simulink model "mcb_pmsm_foc_qep_dyno_f28069m_RAMP_ON_TARGET_R2021b"  (R2021b)
settings: Solver=FixedStepDiscrete  StartTime=0.0  StopTime=4  RelTol=1e-3  EnableMultiTasking=on
InitFcn:
  | mcb_pmsm_foc_qep_dyno_f28069m_data;
undefined symbols (not defined in the file): BaseRPM, DiscIntNeverNeededParam, Down, GPTRIP1SEL, GPTRIP2SEL, inverter_motor1, inverter_motor2, PI_params_motor1, PI_params_motor2, pmsm_motor1, pmsm_motor2, PU_System_motor2, target, Ts, Ts_motor, Ts_speed, TZ1, TZ2, Up
libraries: c2802xlib x10, simulink x10, mcbcontrolslib x8, c280xlib x8, mcbpositiondecoderlib x6, c2806xlib x5, svdschedulerlib x3, autolibpmsmexterior x2, mcbplantlib x2, demo_controls x1, hdlsllib x1, slpidlib x1
(part 2 of 3)

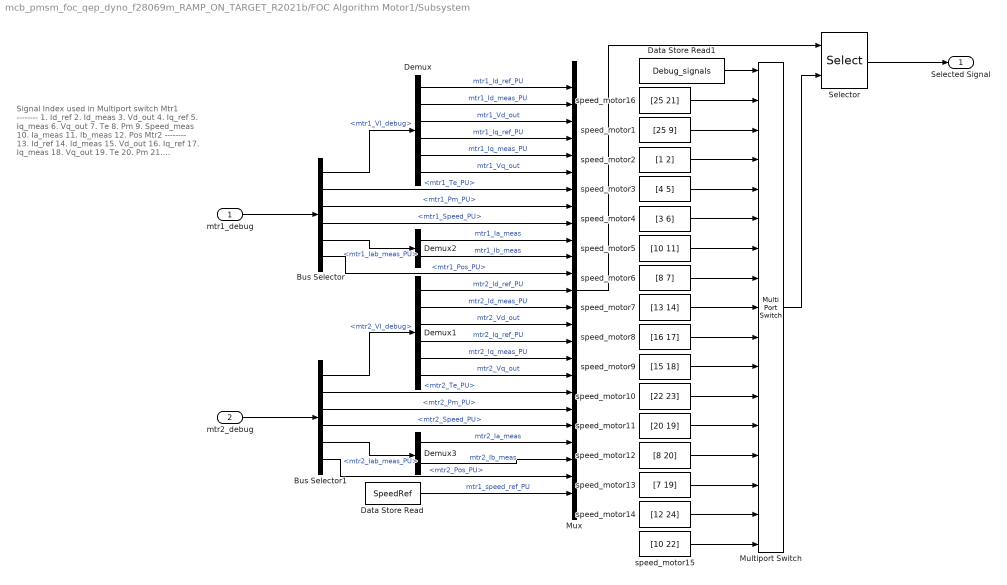
== system mcb_pmsm_foc_qep_dyno_f28069m_RAMP_ON_TARGET_R2021b/FOC Algorithm Motor1/Subsystem ==
  note: Signal Index used in Multiport switch
      | Mtr1
      | --------
      | 1. Id_ref
      | 2. Id_meas
      | 3. Vd_out
      | 4. Iq_ref
      | 5. Iq_meas
      | 6. Vq_out
      | 7. Te
      | 8. Pm
      | 9. Speed_meas
      | 10. Ia_meas
      | 11. Ib_meas
      | 12. Pos
      |
      | Mtr2
      | --------
      | 13. Id_ref
      | 14. Id_meas
      | 15. Vd_out
      | 16. Iq_ref
      | 17. Iq_meas
      | 18. Vq_out
      | 19. Te
      | 20. Pm
      | 21. Speed_meas
      | 22. Ia_meas
      | 23. Ib_meas
      | 24. Pos
      |
      | 25.Speed ref
  mtr1_debug : Inport
  mtr2_debug : Inport  Port=2
  Bus Selector : BusSelector  OutputSignals=mtr1_VI_debug,mtr1_Te_PU,mtr1_Pm_PU,mtr1_Speed_PU,mtr1_Iab_meas_PU,mtr1_Pos_PU
  Bus Selector1 : BusSelector  OutputSignals=mtr2_VI_debug,mtr2_Te_PU,mtr2_Pm_PU,mtr2_Speed_PU,mtr2_Iab_meas_PU,mtr2_Pos_PU
  Data Store Read : DataStoreRead  DataStoreName=SpeedRef  IndexOptions=Index vector (dialog)  Indices=1  OutputSizes=1
  Data Store Read1 : DataStoreRead  DataStoreName=Debug_signals  IndexOptions=Index vector (dialog)  Indices=1  OutputSizes=1
  Demux : Demux  Outputs=6
  Demux1 : Demux  Outputs=6
  Demux2 : Demux  Outputs=2
  Demux3 : Demux  Outputs=2
  Multiport Switch : MultiPortSwitch  DataPortOrder=Zero-based contiguous  Inputs=16  DiagnosticForDefault=Warning  zeroidx=on  OutDataTypeStr=uint16  RndMeth=Simplest
  Mux : Mux  Inputs=25
  Selector : Selector  InputPortWidth=25  IndexOptions=Index vector (port)  Indices=[1 3]  OutputSizes=1
  speed_motor1 : Constant  Value=[25 9]  OutDataTypeStr=uint16  SampleTime=-1
  speed_motor10 : Constant  Value=[22 23]  OutDataTypeStr=uint16  SampleTime=-1
  speed_motor11 : Constant  Value=[20 19]  OutDataTypeStr=uint16  SampleTime=-1
  speed_motor12 : Constant  Value=[8 20]  OutDataTypeStr=uint16  SampleTime=-1
  speed_motor13 : Constant  Value=[7 19]  OutDataTypeStr=uint16  SampleTime=-1
  speed_motor14 : Constant  Value=[12 24]  OutDataTypeStr=uint16  SampleTime=-1
  speed_motor15 : Constant  Value=[10 22]  OutDataTypeStr=uint16  SampleTime=-1
  speed_motor16 : Constant  Value=[25 21]  OutDataTypeStr=uint16  SampleTime=-1
  speed_motor2 : Constant  Value=[1 2]  OutDataTypeStr=uint16  SampleTime=-1
  speed_motor3 : Constant  Value=[4 5]  OutDataTypeStr=uint16  SampleTime=-1
  speed_motor4 : Constant  Value=[3 6]  OutDataTypeStr=uint16  SampleTime=-1
  speed_motor5 : Constant  Value=[10 11]  OutDataTypeStr=uint16  SampleTime=-1
  speed_motor6 : Constant  Value=[8 7]  OutDataTypeStr=uint16  SampleTime=-1
  speed_motor7 : Constant  Value=[13 14]  OutDataTypeStr=uint16  SampleTime=-1
  speed_motor8 : Constant  Value=[16 17]  OutDataTypeStr=uint16  SampleTime=-1
  speed_motor9 : Constant  Value=[15 18]  OutDataTypeStr=uint16  SampleTime=-1
  Selected Signal : Outport
  wires:
  mtr1_debug/1 -> Bus Selector/1
  mtr2_debug/1 -> Bus Selector1/1
  Bus Selector/1 -> Demux/1  "<mtr1_VI_debug>"
  Bus Selector1/1 -> Demux1/1  "<mtr2_VI_debug>"
  Demux/1 -> Mux/1  "mtr1_Id_ref_PU"
  Demux/2 -> Mux/2  "mtr1_Id_meas_PU"
  Demux/3 -> Mux/3  "mtr1_Vd_out"
  Demux/4 -> Mux/4  "mtr1_Iq_ref_PU"
  Demux/5 -> Mux/5  "mtr1_Iq_meas_PU"
  Demux/6 -> Mux/6  "mtr1_Vq_out"
  Bus Selector/2 -> Mux/7  "<mtr1_Te_PU>"
  Bus Selector/3 -> Mux/8  "<mtr1_Pm_PU>"
  Bus Selector/4 -> Mux/9  "<mtr1_Speed_PU>"
  Bus Selector/5 -> Demux2/1  "<mtr1_Iab_meas_PU>"
  Bus Selector/6 -> Mux/12  "<mtr1_Pos_PU>"
  Demux1/1 -> Mux/13  "mtr2_Id_ref_PU"
  Demux1/2 -> Mux/14  "mtr2_Id_meas_PU"
  Demux1/3 -> Mux/15  "mtr2_Vd_out"
  Demux1/4 -> Mux/16  "mtr2_Iq_ref_PU"
  Demux1/5 -> Mux/17  "mtr2_Iq_meas_PU"
  Demux1/6 -> Mux/18  "mtr2_Vq_out"
  Bus Selector1/2 -> Mux/19  "<mtr2_Te_PU>"
  Bus Selector1/3 -> Mux/20  "<mtr2_Pm_PU>"
  Bus Selector1/4 -> Mux/21  "<mtr2_Speed_PU>"
  Bus Selector1/5 -> Demux3/1  "<mtr2_Iab_meas_PU>"
  Bus Selector1/6 -> Mux/24  "<mtr2_Pos_PU>"
  Data Store Read/1 -> Mux/25  "mtr1_speed_ref_PU"
  Mux/1 -> Selector/1
  Data Store Read1/1 -> Multiport Switch/1
  Multiport Switch/1 -> Selector/2
  Selector/1 -> Selected Signal/1
  Demux2/1 -> Mux/10  "mtr1_Ia_meas"
  Demux2/2 -> Mux/11  "mtr1_Ib_meas"
  Demux3/1 -> Mux/22  "mtr2_Ia_meas"
  Demux3/2 -> Mux/23  "mtr2_Ib_meas"
  speed_motor1/1 -> Multiport Switch/3
  speed_motor2/1 -> Multiport Switch/4
  speed_motor3/1 -> Multiport Switch/5
  speed_motor4/1 -> Multiport Switch/6
  speed_motor5/1 -> Multiport Switch/7
  speed_motor6/1 -> Multiport Switch/8
  speed_motor7/1 -> Multiport Switch/9
  speed_motor8/1 -> Multiport Switch/10
  speed_motor9/1 -> Multiport Switch/11
  speed_motor10/1 -> Multiport Switch/12
  speed_motor11/1 -> Multiport Switch/13
  speed_motor12/1 -> Multiport Switch/14
  speed_motor13/1 -> Multiport Switch/15
  speed_motor14/1 -> Multiport Switch/16
  speed_motor15/1 -> Multiport Switch/17
  speed_motor16/1 -> Multiport Switch/2

== system mcb_pmsm_foc_qep_dyno_f28069m_RAMP_ON_TARGET_R2021b/FOC Algorithm Motor2/Control_System ==
  Iab_meas_PU : Inport
  Pos_PU : Inport  Port=2
  EnClosedLoop : Inport  Port=3
  Idq_ref_PU : Inport  Port=4
  Closed loop : Subsystem
  Constant : Constant  Value=0  OutDataTypeStr=dataType
  Mux1 : Mux  Inputs=3
  Switch : Switch  Criteria=u2 > Threshold  Threshold=0.5
  Duty_Cycles : Outport  VectorParamsAs1DForOutWhenUnconnected=off
  Out2 : Outport  Port=2
  wires:
  EnClosedLoop/1 -> Closed loop/4(EnablePWM), Closed loop/Enable, Switch/2
  Switch/1 -> Duty_Cycles/1
  Idq_ref_PU/1 -> Closed loop/3(Idq_ref_PU)
  Pos_PU/1 -> Closed loop/2(Pos_PU)
  Iab_meas_PU/1 -> Closed loop/1(Iab_meas_PU)
  Mux1/1 -> Switch/3
  Constant/1 -> Mux1/3, Mux1/2, Mux1/1
  Closed loop/1(Vabc in PU) -> Switch/1
  Closed loop/2(Idq_debug) -> Out2/1

== system mcb_pmsm_foc_qep_dyno_f28069m_RAMP_ON_TARGET_R2021b/FOC Algorithm Motor2/Enable Motor2 after a delay ==
  Delay to start motor1 (codegen) : Subsystem  TreatAsAtomicUnit=on  VariantControl=(codegen)
  Delay to start motor2 (sim) : Subsystem  VariantControl=(sim)

== system mcb_pmsm_foc_qep_dyno_f28069m_RAMP_ON_TARGET_R2021b/FOC Algorithm Motor2/HW_Inputs1 ==
  Sim : Inport
  Sensor Driver Blocks (codegen) : Subsystem  VariantControl=(codegen)
  Sensor Driver Blocks (sim) : Subsystem  VariantControl=(sim)
  out : Outport

== system mcb_pmsm_foc_qep_dyno_f28069m_RAMP_ON_TARGET_R2021b/FOC Algorithm Motor2/Input Scaling ==
  note: Current Measurements
  Ia_ADC : Inport
  Ib_ADC : Inport  Port=2
  QEP_Position_Count : Inport  Port=3
  QEP_Index_Latch : Inport  Port=4
  " Calculate Speed" : Subsystem
  Calculate Phase Currents : Subsystem
  Constant : Constant  Value=pmsm_motor2.PositionOffset  OutDataTypeStr=dataType  SampleTime=-1
  speed_PU : Outport
  Iab_meas_PU : Outport  Port=2
  Pos_PU : Outport  Port=3
  EnClosedLoop : Outport  Port=4
  wires:
  " Calculate Speed"/2(speed) -> speed_PU/1
  Calculate Phase Currents/1(Iab_meas_PU) -> Iab_meas_PU/1  "Iab_fb_PU"
  QEP_Position_Count/1 -> " Calculate Speed"/1(QEP_Position_Count)
  " Calculate Speed"/1(Theta_e) -> Pos_PU/1
  Ia_ADC/1 -> Calculate Phase Currents/1(Ia_ADC)
  Ib_ADC/1 -> Calculate Phase Currents/2(Ib_ADC)
  Constant/1 -> " Calculate Speed"/3(Offset)
  QEP_Index_Latch/1 -> " Calculate Speed"/2(QEP_Index_Latch)
  " Calculate Speed"/3(IndexFound) -> EnClosedLoop/1

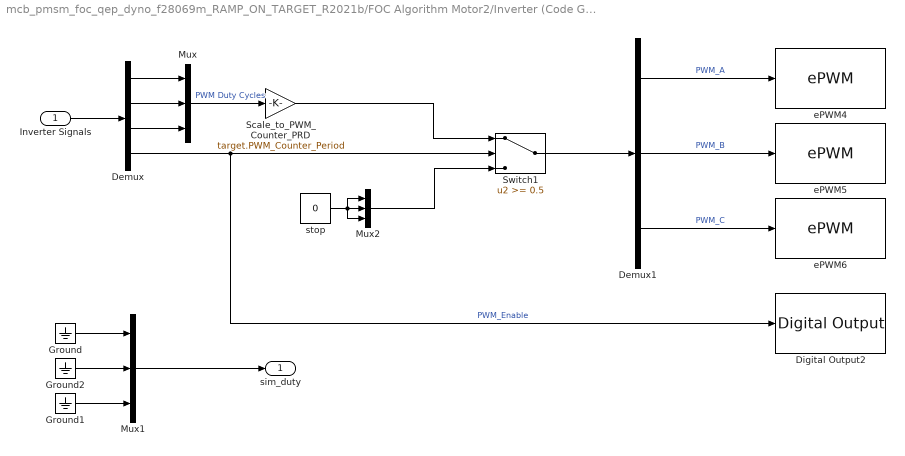
== system mcb_pmsm_foc_qep_dyno_f28069m_RAMP_ON_TARGET_R2021b/FOC Algorithm Motor2/Inverter (Code Generation) ==
  Inverter Signals : Inport
  Demux : Demux
  Demux1 : Demux  Outputs=3
  Digital Output2 : c2806xlib/Digital Output  GPIO_Number=GPIO50~GPIO55  GPIO_Bit0=off  GPIO_BIT0_Toggle=off  GPIO_Bit1=off  GPIO_BIT1_Toggle=off  GPIO_Bit2=off  GPIO_BIT2_Toggle=off  GPIO_Bit3=off  GPIO_BIT3_Toggle=off  GPIO_Bit4=on  GPIO_BIT4_Toggle=off  GPIO_Bit5=off  GPIO_BIT5_Toggle=off  GPIO_Bit6=off  GPIO_BIT6_Toggle=off  GPIO_Bit7=off  GPIO_BIT7_Toggle=off
  Ground : Ground
  Ground1 : Ground
  Ground2 : Ground
  Mux : Mux  Inputs=3
  Mux1 : Mux  Inputs=3
  Mux2 : Mux  Inputs=3
  Scale_to_PWM_Counter_PRD : Gain  Gain=target.PWM_Counter_Period  OutDataTypeStr=uint16  RndMeth=Simplest
  Switch1 : Switch  Threshold=0.5
  ePWM4 : c2802xlib/ePWM  PwmType=C2000  useModule=ePWM4  ePWMxLINKTBPRD=Not Linked  periodUnits=Clock cycles  timerSource=Specify via dialog  timerPeriod_clk=target.PWM_Counter_Period+1  timerPeriod_sec=64000  tbshadow=Counter equals to zero  countingMode=Up-Down  phaseActiveEnable=Set counter to phase value specified via dialog  phaseDirection=Count down after sync  phaseActive=target.PWM_Counter_Period+1  synchronizationEnable=off  dcaevt1Sync=off  dcbevt1Sync=off  synchronizationOption=Pass through (EPWMxSYNCI or SWFSYNC)  dcbevt1SyncOut=off  dcaevt1SyncOut=off  cmpdSyncOut=off  cmpcSyncOut=off  cmpbSyncOut=off  zeroSyncOut=off  swfSyncOut=on  perSynchronizationOption=Counter equals to period (CTR=PRD)  clockPrescale=1  HSclockPrescale=1  enswap=off  ePWMxAStatus=on  ePWMxAactionLogic1=Do nothing  ePWMxAactionLogic2=Do nothing  ePWMxAactionLogic3=Clear  ePWMxAactionLogic4=Set  ePWMxAactionLogic5=Do nothing  ePWMxAactionLogic6=Do nothing  ePWMxACSFenable=off  ePWMxACSFvalue=Forcing disable  ePWMxASFreload=Zero  ePWMxBStatus=off  ePWMxBactionLogic1=Do nothing  ePWMxBactionLogic2=Set  ePWMxBactionLogic3=Do nothing  ePWMxBactionLogic4=Do nothing  ePWMxBactionLogic5=Clear  ePWMxBactionLogic6=Do nothing  ePWMxBCSFenable=off  ePWMxBCSFvalue=Forcing disable  ePWMxBSFreload=Zero  ePWNxBOutWay=off  ePWMxLINKCMPA=Not Linked  CMPAUnits=Clock cycles  CMPASource=Input port  CMPAValue_per=32000  CMPAValue_clk=target.PWM_Counter_Period/2+1  enCMPAshadow=Counter equals to zero (CTR=Zero)  ePWMxLINKCMPB=Not Linked  CMPBUnits=Clock cycles  CMPBSource=Specify via dialog  CMPBValue_per=50  CMPBValue_clk=target.PWM_Counter_Period/2+1  enCMPBshadow=Counter equals to zero (CTR=Zero)  ePWMxLINKCMPC=Not Linked  CMPCUnits=Clock cycles  CMPCSource=Specify via dialog  CMPCValue_per=50  CMPCValue_clk=32000  enCMPCshadow=Counter equals to zero (CTR=Zero)  ePWMxLINKCMPD=Not Linked  CMPDUnits=Clock cycles  CMPDSource=Specify via dialog  CMPDValue_per=50  CMPDValue_clk=32000  enCMPDshadow=Counter equals to zero (CTR=Zero)  enableDBePWMxA=on  enableDBePWMxB=on  enhalfcycle=off  DBpolarity=Active high complementary (AHC)  DBedgeDelay=Positive  DBSource_ePWMxA=ePWMxA  DBSource_ePWMxB=ePWMxA  DBPeriodUnits=Clock cycles  DBperiodSource=Specify via dialog  REDperiod=15  FEDperiod=15  REDperiod_sec=0  FEDperiod_sec=0  LoadModeDBRED=Immediate without using shadow  LoadModeDBFED=Immediate without using shadow  adcstartModuleA=on  adcrequestEventA=First event  adcstartEventA=Counter equals to period (CTR=PRD)  adcstartEventA_type2=Digital Compare Module A Event 1 start of conversion (DCAEVT1.soc)  adcstartModuleB=off  adcrequestEventB=First event  adcstartEventB=Counter equals to zero (CTR=Zero)  adcstartEventB_type2=Counter equals to zero (CTR=Zero)  intEn=off  intPrd=First event  intSel=Counter equals to zero (CTR=Zero)  intSel_type2=Counter equals to zero (CTR=Zero)  hrpe=off  enHRPWM=off  HRPWM_LoadMode=Counter equals to period (CTR=PRD)  HRPWM_CTLMode=Duty or Period control mode  HRPWM_EDGMode=Both edge  hrpeb=off  enHRPWMB=off  HRPWM_LoadModeB=Counter equals to zero (CTR=ZERO)  HRPWM_CTLModeB=Duty or Period control mode  HRPWM_EDGModeB=Both edge  enHRDBRED=off  enHRDBFED=off  enSFO=on  enautoconv=on  chopperEnable=off  chopperFrequency=1  chopperFirstwidth=1  chopperDuty=12.5%  tripZonesource=Specify via dialog  tzselOSHT1=off  tzselOSHT2=off  tzselOSHT3=off  tzselOSHDCAEV1=off  tzselOSHDCBEV1=off  tzselCBC1=off  tzselCBC2=off  tzselCBC3=off  tzselCBCDCAEV2=off  tzselCBCDCBEV2=off  tzselOSHT4=off  tzselOSHT5=off  tzselOSHT6=off  tzselCBC4=off  tzselCBC5=off  tzselCBC6=off  enTzOstIntr=off  enTzCbcIntr=off  enTzDCAEVT1Intr=off  enTzDCAEVT2Intr=off  enTzDCBEVT1Intr=off  enTzDCBEVT2Intr=off  ePWMxAforced=No action  ePWMxBforced=No action  DCAEVT1forced=No action  DCBEVT1forced=No action  DCAEVT2forced=No action  DCBEVT2forced=No action  dcah=Trip Zone 1 input (TZ1)  dcal=Trip Zone 2 input (TZ2)  dcbh=Trip Zone 1 input (TZ1)  dcbl=Trip Zone 2 input (TZ2)  dcah_type2=GPTRIP1SEL/(TZ1)  dcal_type2=GPTRIP2SEL/(TZ2)  dcbh_type2=GPTRIP1SEL/(TZ1)  dcbl_type2=GPTRIP2SEL/(TZ2)  gendcaevt1=Event disabled  gendcaevt2=Event disabled  gendcbevt1=Event disabled  gendcbevt2=Event disabled  dcaevt1src=DCAEVT1 with sync  dcaevt2src=DCAEVT2 with sync  dcbevt1src=DCBEVT1 with sync  dcbevt2src=DCBEVT2 with sync  pulsesel=Counter equals to zero (CTR=Zero)  blankinv=off  blankoffset=0  blankwidth=0  evsrcsel=Filtered version of DCAEVT1 (DCAEVT1FILT)  encape=off
  ePWM5 : c2802xlib/ePWM  PwmType=C2000  useModule=ePWM5  ePWMxLINKTBPRD=Not Linked  periodUnits=Clock cycles  timerSource=Specify via dialog  timerPeriod_clk=target.PWM_Counter_Period+1  timerPeriod_sec=64000  tbshadow=Counter equals to zero  countingMode=Up-Down  phaseActiveEnable=Set counter to phase value specified via dialog  phaseDirection=Count down after sync  phaseActive=target.PWM_Counter_Period+1  synchronizationEnable=off  dcaevt1Sync=off  dcbevt1Sync=off  synchronizationOption=Pass through (EPWMxSYNCI or SWFSYNC)  dcbevt1SyncOut=off  dcaevt1SyncOut=off  cmpdSyncOut=off  cmpcSyncOut=off  cmpbSyncOut=off  zeroSyncOut=off  swfSyncOut=on  perSynchronizationOption=Counter equals to period (CTR=PRD)  clockPrescale=1  HSclockPrescale=1  enswap=off  ePWMxAStatus=on  ePWMxAactionLogic1=Do nothing  ePWMxAactionLogic2=Do nothing  ePWMxAactionLogic3=Clear  ePWMxAactionLogic4=Set  ePWMxAactionLogic5=Do nothing  ePWMxAactionLogic6=Do nothing  ePWMxACSFenable=off  ePWMxACSFvalue=Forcing disable  ePWMxASFreload=Zero  ePWMxBStatus=off  ePWMxBactionLogic1=Do nothing  ePWMxBactionLogic2=Set  ePWMxBactionLogic3=Do nothing  ePWMxBactionLogic4=Do nothing  ePWMxBactionLogic5=Clear  ePWMxBactionLogic6=Do nothing  ePWMxBCSFenable=off  ePWMxBCSFvalue=Forcing disable  ePWMxBSFreload=Zero  ePWNxBOutWay=off  ePWMxLINKCMPA=Not Linked  CMPAUnits=Clock cycles  CMPASource=Input port  CMPAValue_per=32000  CMPAValue_clk=target.PWM_Counter_Period/2+1  enCMPAshadow=Counter equals to zero (CTR=Zero)  ePWMxLINKCMPB=Not Linked  CMPBUnits=Clock cycles  CMPBSource=Specify via dialog  CMPBValue_per=50  CMPBValue_clk=target.PWM_Counter_Period/2+1  enCMPBshadow=Counter equals to zero (CTR=Zero)  ePWMxLINKCMPC=Not Linked  CMPCUnits=Clock cycles  CMPCSource=Specify via dialog  CMPCValue_per=50  CMPCValue_clk=32000  enCMPCshadow=Counter equals to zero (CTR=Zero)  ePWMxLINKCMPD=Not Linked  CMPDUnits=Clock cycles  CMPDSource=Specify via dialog  CMPDValue_per=50  CMPDValue_clk=32000  enCMPDshadow=Counter equals to zero (CTR=Zero)  enableDBePWMxA=on  enableDBePWMxB=on  enhalfcycle=off  DBpolarity=Active high complementary (AHC)  DBedgeDelay=Positive  DBSource_ePWMxA=ePWMxA  DBSource_ePWMxB=ePWMxA  DBPeriodUnits=Clock cycles  DBperiodSource=Specify via dialog  REDperiod=15  FEDperiod=15  REDperiod_sec=0  FEDperiod_sec=0  LoadModeDBRED=Immediate without using shadow  LoadModeDBFED=Immediate without using shadow  adcstartModuleA=off  adcrequestEventA=First event  adcstartEventA=Digital Compare Module A Event 1 start of conversion (DCAEVT1.soc)  adcstartEventA_type2=Digital Compare Module A Event 1 start of conversion (DCAEVT1.soc)  adcstartModuleB=off  adcrequestEventB=First event  adcstartEventB=Counter equals to zero (CTR=Zero)  adcstartEventB_type2=Counter equals to zero (CTR=Zero)  intEn=off  intPrd=First event  intSel=Counter equals to zero (CTR=Zero)  intSel_type2=Counter equals to zero (CTR=Zero)  hrpe=off  enHRPWM=off  HRPWM_LoadMode=Counter equals to period (CTR=PRD)  HRPWM_CTLMode=Duty or Period control mode  HRPWM_EDGMode=Both edge  hrpeb=off  enHRPWMB=off  HRPWM_LoadModeB=Counter equals to zero (CTR=ZERO)  HRPWM_CTLModeB=Duty or Period control mode  HRPWM_EDGModeB=Both edge  enHRDBRED=off  enHRDBFED=off  enSFO=on  enautoconv=on  chopperEnable=off  chopperFrequency=1  chopperFirstwidth=1  chopperDuty=12.5%  tripZonesource=Specify via dialog  tzselOSHT1=off  tzselOSHT2=off  tzselOSHT3=off  tzselOSHDCAEV1=off  tzselOSHDCBEV1=off  tzselCBC1=off  tzselCBC2=off  tzselCBC3=off  tzselCBCDCAEV2=off  tzselCBCDCBEV2=off  tzselOSHT4=off  tzselOSHT5=off  tzselOSHT6=off  tzselCBC4=off  tzselCBC5=off  tzselCBC6=off  enTzOstIntr=off  enTzCbcIntr=off  enTzDCAEVT1Intr=off  enTzDCAEVT2Intr=off  enTzDCBEVT1Intr=off  enTzDCBEVT2Intr=off  ePWMxAforced=No action  ePWMxBforced=No action  DCAEVT1forced=No action  DCBEVT1forced=No action  DCAEVT2forced=No action  DCBEVT2forced=No action  dcah=Trip Zone 1 input (TZ1)  dcal=Trip Zone 2 input (TZ2)  dcbh=Trip Zone 1 input (TZ1)  dcbl=Trip Zone 2 input (TZ2)  dcah_type2=GPTRIP1SEL/(TZ1)  dcal_type2=GPTRIP2SEL/(TZ2)  dcbh_type2=GPTRIP1SEL/(TZ1)  dcbl_type2=GPTRIP2SEL/(TZ2)  gendcaevt1=Event disabled  gendcaevt2=Event disabled  gendcbevt1=Event disabled  gendcbevt2=Event disabled  dcaevt1src=DCAEVT1 with sync  dcaevt2src=DCAEVT2 with sync  dcbevt1src=DCBEVT1 with sync  dcbevt2src=DCBEVT2 with sync  pulsesel=Counter equals to zero (CTR=Zero)  blankinv=off  blankoffset=0  blankwidth=0  evsrcsel=Filtered version of DCAEVT1 (DCAEVT1FILT)  encape=off
  ePWM6 : c2802xlib/ePWM  PwmType=C2000  useModule=ePWM6  ePWMxLINKTBPRD=Not Linked  periodUnits=Clock cycles  timerSource=Specify via dialog  timerPeriod_clk=target.PWM_Counter_Period+1  timerPeriod_sec=64000  tbshadow=Counter equals to zero  countingMode=Up-Down  phaseActiveEnable=Set counter to phase value specified via dialog  phaseDirection=Count down after sync  phaseActive=target.PWM_Counter_Period+1  synchronizationEnable=off  dcaevt1Sync=off  dcbevt1Sync=off  synchronizationOption=Disable  dcbevt1SyncOut=off  dcaevt1SyncOut=off  cmpdSyncOut=off  cmpcSyncOut=off  cmpbSyncOut=off  zeroSyncOut=off  swfSyncOut=off  perSynchronizationOption=Counter equals to period (CTR=PRD)  clockPrescale=1  HSclockPrescale=1  enswap=off  ePWMxAStatus=on  ePWMxAactionLogic1=Do nothing  ePWMxAactionLogic2=Do nothing  ePWMxAactionLogic3=Clear  ePWMxAactionLogic4=Set  ePWMxAactionLogic5=Do nothing  ePWMxAactionLogic6=Do nothing  ePWMxACSFenable=off  ePWMxACSFvalue=Forcing disable  ePWMxASFreload=Zero  ePWMxBStatus=off  ePWMxBactionLogic1=Do nothing  ePWMxBactionLogic2=Set  ePWMxBactionLogic3=Do nothing  ePWMxBactionLogic4=Do nothing  ePWMxBactionLogic5=Clear  ePWMxBactionLogic6=Do nothing  ePWMxBCSFenable=off  ePWMxBCSFvalue=Forcing disable  ePWMxBSFreload=Zero  ePWNxBOutWay=off  ePWMxLINKCMPA=Not Linked  CMPAUnits=Clock cycles  CMPASource=Input port  CMPAValue_per=32000  CMPAValue_clk=target.PWM_Counter_Period/2+1  enCMPAshadow=Counter equals to zero (CTR=Zero)  ePWMxLINKCMPB=Not Linked  CMPBUnits=Clock cycles  CMPBSource=Specify via dialog  CMPBValue_per=50  CMPBValue_clk=target.PWM_Counter_Period/2+1  enCMPBshadow=Counter equals to zero (CTR=Zero)  ePWMxLINKCMPC=Not Linked  CMPCUnits=Clock cycles  CMPCSource=Specify via dialog  CMPCValue_per=50  CMPCValue_clk=32000  enCMPCshadow=Counter equals to zero (CTR=Zero)  ePWMxLINKCMPD=Not Linked  CMPDUnits=Clock cycles  CMPDSource=Specify via dialog  CMPDValue_per=50  CMPDValue_clk=32000  enCMPDshadow=Counter equals to zero (CTR=Zero)  enableDBePWMxA=on  enableDBePWMxB=on  enhalfcycle=off  DBpolarity=Active high complementary (AHC)  DBedgeDelay=Positive  DBSource_ePWMxA=ePWMxA  DBSource_ePWMxB=ePWMxA  DBPeriodUnits=Clock cycles  DBperiodSource=Specify via dialog  REDperiod=15  FEDperiod=15  REDperiod_sec=0  FEDperiod_sec=0  LoadModeDBRED=Immediate without using shadow  LoadModeDBFED=Immediate without using shadow  adcstartModuleA=off  adcrequestEventA=First event  adcstartEventA=Digital Compare Module A Event 1 start of conversion (DCAEVT1.soc)  adcstartEventA_type2=Digital Compare Module A Event 1 start of conversion (DCAEVT1.soc)  adcstartModuleB=off  adcrequestEventB=First event  adcstartEventB=Counter equals to zero (CTR=Zero)  adcstartEventB_type2=Counter equals to zero (CTR=Zero)  intEn=off  intPrd=First event  intSel=Counter equals to zero (CTR=Zero)  intSel_type2=Counter equals to zero (CTR=Zero)  hrpe=off  enHRPWM=off  HRPWM_LoadMode=Counter equals to period (CTR=PRD)  HRPWM_CTLMode=Duty or Period control mode  HRPWM_EDGMode=Both edge  hrpeb=off  enHRPWMB=off  HRPWM_LoadModeB=Counter equals to zero (CTR=ZERO)  HRPWM_CTLModeB=Duty or Period control mode  HRPWM_EDGModeB=Both edge  enHRDBRED=off  enHRDBFED=off  enSFO=on  enautoconv=on  chopperEnable=off  chopperFrequency=1  chopperFirstwidth=1  chopperDuty=12.5%  tripZonesource=Specify via dialog  tzselOSHT1=off  tzselOSHT2=off  tzselOSHT3=off  tzselOSHDCAEV1=off  tzselOSHDCBEV1=off  tzselCBC1=off  tzselCBC2=off  tzselCBC3=off  tzselCBCDCAEV2=off  tzselCBCDCBEV2=off  tzselOSHT4=off  tzselOSHT5=off  tzselOSHT6=off  tzselCBC4=off  tzselCBC5=off  tzselCBC6=off  enTzOstIntr=off  enTzCbcIntr=off  enTzDCAEVT1Intr=off  enTzDCAEVT2Intr=off  enTzDCBEVT1Intr=off  enTzDCBEVT2Intr=off  ePWMxAforced=No action  ePWMxBforced=No action  DCAEVT1forced=No action  DCBEVT1forced=No action  DCAEVT2forced=No action  DCBEVT2forced=No action  dcah=Trip Zone 1 input (TZ1)  dcal=Trip Zone 2 input (TZ2)  dcbh=Trip Zone 1 input (TZ1)  dcbl=Trip Zone 2 input (TZ2)  dcah_type2=GPTRIP1SEL/(TZ1)  dcal_type2=GPTRIP2SEL/(TZ2)  dcbh_type2=GPTRIP1SEL/(TZ1)  dcbl_type2=GPTRIP2SEL/(TZ2)  gendcaevt1=Event disabled  gendcaevt2=Event disabled  gendcbevt1=Event disabled  gendcbevt2=Event disabled  dcaevt1src=DCAEVT1 with sync  dcaevt2src=DCAEVT2 with sync  dcbevt1src=DCBEVT1 with sync  dcbevt2src=DCBEVT2 with sync  pulsesel=Counter equals to zero (CTR=Zero)  blankinv=off  blankoffset=0  blankwidth=0  evsrcsel=Filtered version of DCAEVT1 (DCAEVT1FILT)  encape=off
  stop : Constant  Value=0  OutDataTypeStr=uint16
  sim_duty : Outport  VectorParamsAs1DForOutWhenUnconnected=off
  wires:
  Demux1/3 -> ePWM6/1  "PWM_C"
  Scale_to_PWM_Counter_PRD/1 -> Switch1/1
  Mux2/1 -> Switch1/3
  stop/1 -> Mux2/3, Mux2/2, Mux2/1
  Demux/4 -> Digital Output2/1, Switch1/2  "PWM_Enable"
  Inverter Signals/1 -> Demux/1
  Demux1/2 -> ePWM5/1  "PWM_B"
  Switch1/1 -> Demux1/1
  Demux1/1 -> ePWM4/1  "PWM_A"
  Mux/1 -> Scale_to_PWM_Counter_PRD/1  "PWM Duty Cycles"
  Ground/1 -> Mux1/1
  Ground1/1 -> Mux1/3
  Ground2/1 -> Mux1/2
  Mux1/1 -> sim_duty/1
  Demux/1 -> Mux/1
  Demux/2 -> Mux/2
  Demux/3 -> Mux/3

== system mcb_pmsm_foc_qep_dyno_f28069m_RAMP_ON_TARGET_R2021b/FOC Algorithm Motor2/Inverter (Simulation) ==
  Inverter Signals : Inport
  Data Type Duplicate : DataTypeDuplicate
  Demux : Demux
  Mux : Mux  Inputs=3
  Mux2 : Mux  Inputs=3
  Switch1 : Switch  Threshold=0.5  RndMeth=Simplest
  stop : Constant  Value=0  OutDataTypeStr=Inherit: Inherit via back propagation
  Sim_duty : Outport  VectorParamsAs1DForOutWhenUnconnected=off
  wires:
  Demux/3 -> Mux/3
  Demux/2 -> Mux/2
  Demux/1 -> Mux/1
  Mux/1 -> Switch1/1, Data Type Duplicate/1  "PWM Duty Cycles"
  Demux/4 -> Switch1/2  "PWM Enable"
  Inverter Signals/1 -> Demux/1
  Switch1/1 -> Sim_duty/1
  Mux2/1 -> Switch1/3
  stop/1 -> Mux2/2, Mux2/3, Mux2/1, Data Type Duplicate/2

== system mcb_pmsm_foc_qep_dyno_f28069m_RAMP_ON_TARGET_R2021b/FOC Algorithm Motor2/Output Scaling ==
  Vabc_ref : Inport
  Constant : Constant  Value=0.5  OutDataTypeStr=dataType  SampleTime=-1
  Data Type Conversion : DataTypeConversion  OutDataTypeStr=dataType
  Enable : DataStoreRead  DataStoreName=EnMtr2TrqCtrl  IndexOptions=Index vector (dialog)  Indices=1  OutputSizes=1
  One_by_Two : Gain  Gain=0.5  RndMeth=Simplest  OutDataTypeStr=Inherit: Same as input
  Sum : Sum  Inputs=|++
  PWM_Duty_Cycles : Outport
  PWM_Enable : Outport  Port=2
  wires:
  Data Type Conversion/1 -> PWM_Enable/1
  One_by_Two/1 -> Sum/1
  Enable/1 -> Data Type Conversion/1  "PWM_En"
  Sum/1 -> PWM_Duty_Cycles/1  "Mtr2_PWM_Duty_Cycles"
  Vabc_ref/1 -> One_by_Two/1
  Constant/1 -> Sum/2

== system mcb_pmsm_foc_qep_dyno_f28069m_RAMP_ON_TARGET_R2021b/Hardware Init/HW_Init ==
  HW_Init (Codegen) : Subsystem  VariantControl=(codegen)
  HW_Init (sim) : Subsystem  VariantControl=(sim)

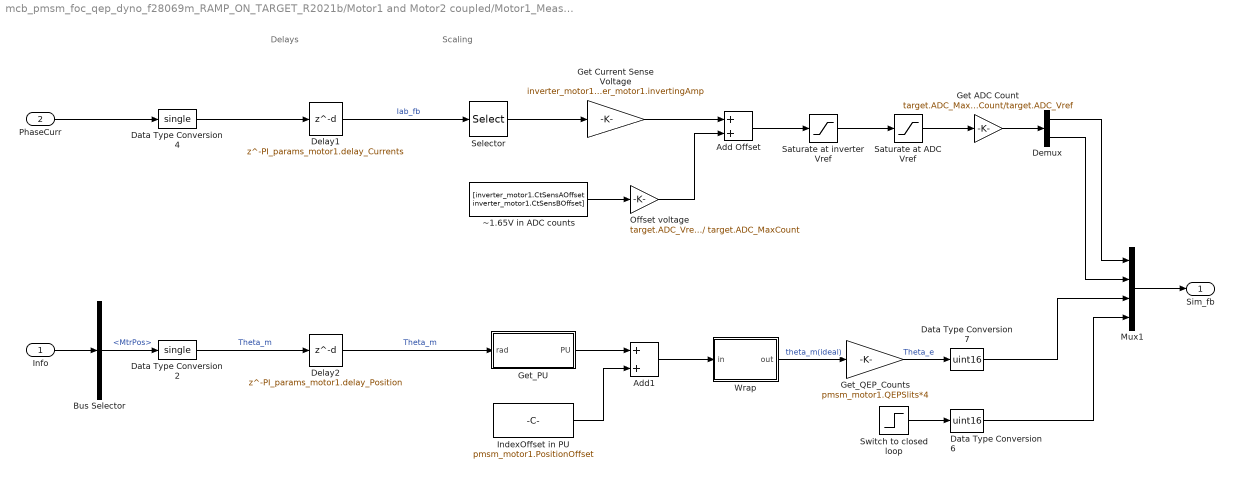
== system mcb_pmsm_foc_qep_dyno_f28069m_RAMP_ON_TARGET_R2021b/Motor1 and Motor2 coupled/Motor1_Measurements ==
  note: Delays
  note: Scaling
  Info : Inport
  PhaseCurr : Inport  Port=2
  Add Offset : Sum  RndMeth=Simplest
  Add1 : Sum  RndMeth=Simplest
  Bus Selector : BusSelector  OutputSignals=MtrPos
  Data Type Conversion2 : DataTypeConversion  OutDataTypeStr=single  RndMeth=Simplest
  Data Type Conversion4 : DataTypeConversion  OutDataTypeStr=single  RndMeth=Simplest
  Data Type Conversion6 : DataTypeConversion  OutDataTypeStr=uint16  RndMeth=Simplest
  Data Type Conversion7 : DataTypeConversion  OutDataTypeStr=uint16  RndMeth=Simplest
  Delay1 : Delay  DelayLength=PI_params_motor1.delay_Currents
  Delay2 : Delay  DelayLength=PI_params_motor1.delay_Position
  Demux : Demux  Outputs=2
  Get ADC Count : Gain  Gain=target.ADC_MaxCount/target.ADC_Vref  OutMin=0  OutMax=target.ADC_MaxCount  OutDataTypeStr=uint16  RndMeth=Simplest
  Get Current Sense Voltage : Gain  Gain=inverter_motor1.ISenseVoltPerAmp * inverter_motor1.invertingAmp  RndMeth=Simplest  OutDataTypeStr=Inherit: Same as input
  "Get_PU " : Subsystem
  Get_QEP_Counts : Gain  Gain=pmsm_motor1.QEPSlits*4  OutDataTypeStr=uint16  RndMeth=Simplest
  IndexOffset in PU : Constant  Value=pmsm_motor1.PositionOffset  OutDataTypeStr=single  SampleTime=-1
  Mux1 : Mux
  Offset voltage : Gain  Gain=target.ADC_Vref / target.ADC_MaxCount  RndMeth=Simplest
  Saturate at ADC Vref : Saturate  UpperLimit=target.ADC_Vref  LowerLimit=0
  Saturate at inverter Vref : Saturate  UpperLimit=inverter_motor1.ISenseVref  LowerLimit=0
  Selector : Selector  InputPortWidth=3  IndexOptions=Index vector (dialog)  Indices=[1 2]  OutputSizes=1
  "Switch to closed loop " : Step  Time=0.1  SampleTime=Ts_motor
  Wrap : Subsystem
  ~1.65V in ADC counts : Constant  Value=[inverter_motor1.CtSensAOffset inverter_motor1.CtSensBOffset]  OutDataTypeStr=uint16  SampleTime=-1
  Sim_fb : Outport  VectorParamsAs1DForOutWhenUnconnected=off
  wires:
  "Switch to closed loop "/1 -> Data Type Conversion6/1
  Data Type Conversion6/1 -> Mux1/4
  Data Type Conversion7/1 -> Mux1/3
  IndexOffset in PU/1 -> Add1/2
  Get_QEP_Counts/1 -> Data Type Conversion7/1  "Theta_e"
  "Get_PU "/1(PU) -> Add1/1
  Wrap/1(out) -> Get_QEP_Counts/1  "theta_m(ideal)"
  Delay2/1 -> "Get_PU "/1(rad)  "Theta_m"
  Add1/1 -> Wrap/1(in)
  Data Type Conversion2/1 -> Delay2/1  "Theta_m"
  Demux/2 -> Mux1/2
  Mux1/1 -> Sim_fb/1
  Demux/1 -> Mux1/1
  Bus Selector/1 -> Data Type Conversion2/1  "<MtrPos>"
  Info/1 -> Bus Selector/1
  PhaseCurr/1 -> Data Type Conversion4/1
  Data Type Conversion4/1 -> Delay1/1
  Delay1/1 -> Selector/1  "Iab_fb"
  Saturate at ADC Vref/1 -> Get ADC Count/1
  Offset voltage/1 -> Add Offset/2
  Selector/1 -> Get Current Sense Voltage/1
  Get ADC Count/1 -> Demux/1
  Saturate at inverter Vref/1 -> Saturate at ADC Vref/1
  Add Offset/1 -> Saturate at inverter Vref/1
  Get Current Sense Voltage/1 -> Add Offset/1
  ~1.65V in ADC counts/1 -> Offset voltage/1

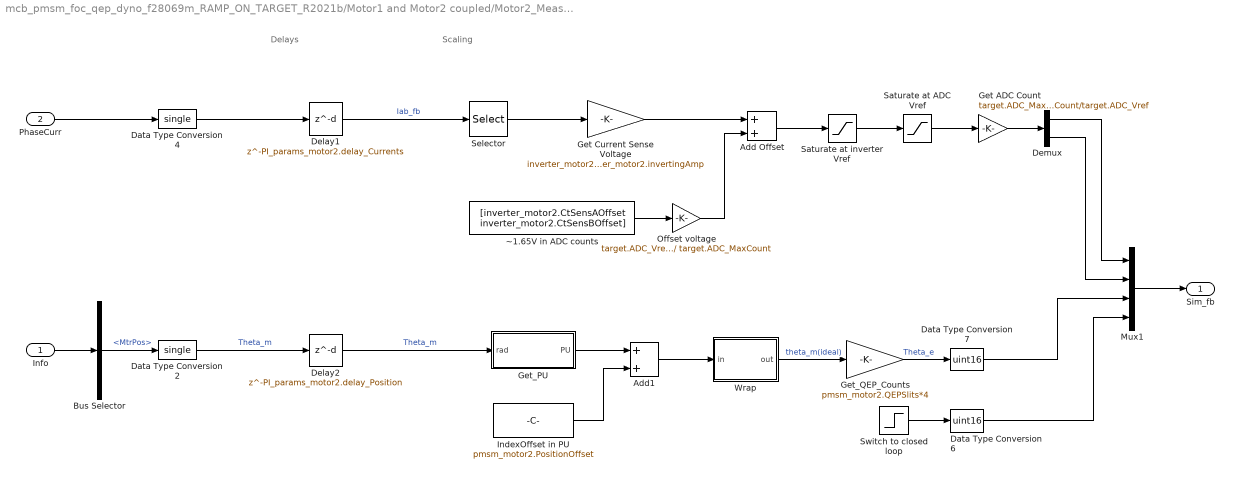
== system mcb_pmsm_foc_qep_dyno_f28069m_RAMP_ON_TARGET_R2021b/Motor1 and Motor2 coupled/Motor2_Measurements ==
  note: Scaling
  note: Delays
  Info : Inport
  PhaseCurr : Inport  Port=2
  Add Offset : Sum  RndMeth=Simplest
  Add1 : Sum  RndMeth=Simplest
  Bus Selector : BusSelector  OutputSignals=MtrPos
  Data Type Conversion2 : DataTypeConversion  OutDataTypeStr=single  RndMeth=Simplest
  Data Type Conversion4 : DataTypeConversion  OutDataTypeStr=single  RndMeth=Simplest
  Data Type Conversion6 : DataTypeConversion  OutDataTypeStr=uint16  RndMeth=Simplest
  Data Type Conversion7 : DataTypeConversion  OutDataTypeStr=uint16  RndMeth=Simplest
  Delay1 : Delay  DelayLength=PI_params_motor2.delay_Currents
  Delay2 : Delay  DelayLength=PI_params_motor2.delay_Position
  Demux : Demux  Outputs=2
  Get ADC Count : Gain  Gain=target.ADC_MaxCount/target.ADC_Vref  OutMin=0  OutMax=target.ADC_MaxCount  OutDataTypeStr=uint16  RndMeth=Simplest
  Get Current Sense Voltage : Gain  Gain=inverter_motor2.ISenseVoltPerAmp * inverter_motor2.invertingAmp  RndMeth=Simplest  OutDataTypeStr=Inherit: Same as input
  "Get_PU " : Subsystem
  Get_QEP_Counts : Gain  Gain=pmsm_motor2.QEPSlits*4  OutDataTypeStr=uint16  RndMeth=Simplest
  IndexOffset in PU : Constant  Value=pmsm_motor2.PositionOffset  OutDataTypeStr=single  SampleTime=-1
  Mux1 : Mux
  Offset voltage : Gain  Gain=target.ADC_Vref / target.ADC_MaxCount  RndMeth=Simplest
  Saturate at ADC Vref : Saturate  UpperLimit=target.ADC_Vref  LowerLimit=0
  Saturate at inverter Vref : Saturate  UpperLimit=inverter_motor2.ISenseVref  LowerLimit=0
  Selector : Selector  InputPortWidth=3  IndexOptions=Index vector (dialog)  Indices=[1 2]  OutputSizes=1
  "Switch to closed loop " : Step  Time=0.1  SampleTime=Ts_motor
  Wrap : Subsystem
  ~1.65V in ADC counts : Constant  Value=[inverter_motor2.CtSensAOffset inverter_motor2.CtSensBOffset]  OutDataTypeStr=uint16  SampleTime=-1
  Sim_fb : Outport  VectorParamsAs1DForOutWhenUnconnected=off
  wires:
  Delay1/1 -> Selector/1  "Iab_fb"
  Data Type Conversion4/1 -> Delay1/1
  PhaseCurr/1 -> Data Type Conversion4/1
  Info/1 -> Bus Selector/1
  Bus Selector/1 -> Data Type Conversion2/1  "<MtrPos>"
  Demux/1 -> Mux1/1
  Mux1/1 -> Sim_fb/1
  Demux/2 -> Mux1/2
  Data Type Conversion2/1 -> Delay2/1  "Theta_m"
  Add1/1 -> Wrap/1(in)
  Delay2/1 -> "Get_PU "/1(rad)  "Theta_m"
  Wrap/1(out) -> Get_QEP_Counts/1  "theta_m(ideal)"
  "Get_PU "/1(PU) -> Add1/1
  Get_QEP_Counts/1 -> Data Type Conversion7/1  "Theta_e"
  IndexOffset in PU/1 -> Add1/2
  Data Type Conversion7/1 -> Mux1/3
  Data Type Conversion6/1 -> Mux1/4
  "Switch to closed loop "/1 -> Data Type Conversion6/1
  Saturate at ADC Vref/1 -> Get ADC Count/1
  Offset voltage/1 -> Add Offset/2
  Selector/1 -> Get Current Sense Voltage/1
  Get ADC Count/1 -> Demux/1
  Saturate at inverter Vref/1 -> Saturate at ADC Vref/1
  Add Offset/1 -> Saturate at inverter Vref/1
  Get Current Sense Voltage/1 -> Add Offset/1
  ~1.65V in ADC counts/1 -> Offset voltage/1

== system mcb_pmsm_foc_qep_dyno_f28069m_RAMP_ON_TARGET_R2021b/Motor1 and Motor2 coupled/Mtr1 Inverter ==
  Duty_abc : Inport
  Average-Value Inverter : mcbplantlib/Average-Value Inverter
  Constant2 : Constant  Value=inverter_motor1.V_dc  OutDataTypeStr=single
  Data Type Conversion1 : DataTypeConversion  OutDataTypeStr=single  RndMeth=Simplest
  Rate Transition3 : RateTransition  Integrity=off  OutPortSampleTime=Ts_inverter
  Vabc : Outport  VectorParamsAs1DForOutWhenUnconnected=off
  wires:
  Constant2/1 -> Average-Value Inverter/2
  Data Type Conversion1/1 -> Rate Transition3/1
  Average-Value Inverter/1 -> Vabc/1
  Duty_abc/1 -> Data Type Conversion1/1
  Rate Transition3/1 -> Average-Value Inverter/1

== system mcb_pmsm_foc_qep_dyno_f28069m_RAMP_ON_TARGET_R2021b/Motor1 and Motor2 coupled/Mtr2 Inverter ==
  Duty_abc : Inport
  Average-Value Inverter : mcbplantlib/Average-Value Inverter
  Constant2 : Constant  Value=inverter_motor2.V_dc  OutDataTypeStr=single
  Data Type Conversion1 : DataTypeConversion  OutDataTypeStr=single  RndMeth=Simplest
  Rate Transition3 : RateTransition  Integrity=off  OutPortSampleTime=Ts_inverter
  Vabc : Outport  VectorParamsAs1DForOutWhenUnconnected=off
  wires:
  Data Type Conversion1/1 -> Rate Transition3/1
  Average-Value Inverter/1 -> Vabc/1
  Duty_abc/1 -> Data Type Conversion1/1
  Rate Transition3/1 -> Average-Value Inverter/1
  Constant2/1 -> Average-Value Inverter/2

== system mcb_pmsm_foc_qep_dyno_f28069m_RAMP_ON_TARGET_R2021b/Serial Receive/Code Generation ==
  SCI Receive : c280xlib/SCI Receive  sciModule=A  dataHead=''  headerCheckMaxCount=16  dataTail=''  dataType=uint16  dataLenOptions=Length via dialog  dataDim=4  maxDataLength=1  initValue=0  errOption=Output the last received value  errValue=0  sampleTime=-1  blockingMode=on  timeOut=0.019444  outputStatus=off
  Data : Outport
  wires:
  SCI Receive/1 -> Data/1

== system mcb_pmsm_foc_qep_dyno_f28069m_RAMP_ON_TARGET_R2021b/Serial Receive/Reference Signal ==
  In1 : Inport
  Data Store Write2 : DataStoreWrite  DataStoreName=Debug_signals  IndexOptions=Index vector (dialog)  Indices=1  OutputSizes=1
  Data_Conditioning : Subsystem
  If : If  IfExpression=u1 == 1  ElseIfExpressions=u1 == 2, u1 == 0  ShowElse=off
  If Action Subsystem : Subsystem  TreatAsAtomicUnit=on
  If Action Subsystem1 : Subsystem  TreatAsAtomicUnit=on
  If Action Subsystem2 : Subsystem  TreatAsAtomicUnit=on
  MATLAB Function : MATLAB Function  TreatAsAtomicUnit=on
  unParse : Subsystem
  Enable_PWM : Outport
  enable : Outport  Port=2
  mode : Outport  Port=3
  slope : Outport  Port=4
  target : Outport  Port=5
  wires:
  If/3 -> If Action Subsystem2/Action
  ? -> Data Store Write2/1
  If/2 -> If Action Subsystem1/Action
  If/1 -> If Action Subsystem/Action
  In1/1 -> Data_Conditioning/1(In1)
  ? -> If/1
  ? -> Enable_PWM/1
  Data_Conditioning/1(ramp_enable) -> MATLAB Function/1(en_in)
  Data_Conditioning/2(target_mode) -> MATLAB Function/2(mode_in)
  Data_Conditioning/4(ramp_slope_rpmps) -> MATLAB Function/3(slope_in)
  Data_Conditioning/5(target_rpm) -> MATLAB Function/4(target_in)
  MATLAB Function/4(target) -> target/1
  MATLAB Function/3(slope) -> slope/1
  MATLAB Function/2(mode) -> mode/1
  MATLAB Function/1(enable) -> enable/1

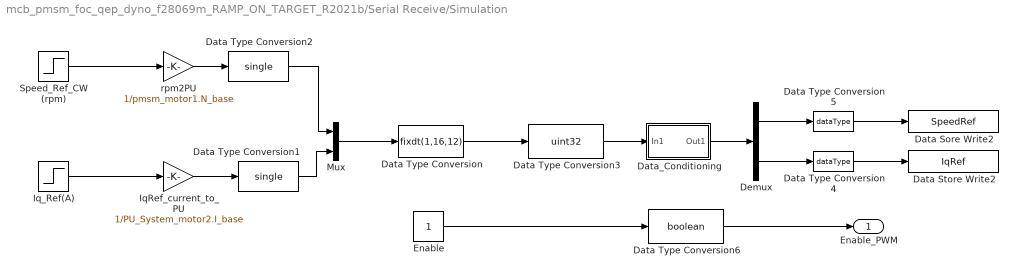
== system mcb_pmsm_foc_qep_dyno_f28069m_RAMP_ON_TARGET_R2021b/Serial Receive/Simulation ==
  Data Sore Write2 : DataStoreWrite  DataStoreName=SpeedRef  IndexOptions=Index vector (dialog)  Indices=1  OutputSizes=1
  Data Store Write2 : DataStoreWrite  DataStoreName=IqRef  IndexOptions=Index vector (dialog)  Indices=1  OutputSizes=1
  Data Type Conversion : DataTypeConversion  OutDataTypeStr=fixdt(1,16,12)  RndMeth=Simplest
  Data Type Conversion1 : DataTypeConversion  OutDataTypeStr=single  RndMeth=Simplest
  Data Type Conversion2 : DataTypeConversion  OutDataTypeStr=single  RndMeth=Simplest
  Data Type Conversion3 : DataTypeConversion  OutDataTypeStr=uint32  ConvertRealWorld=Stored Integer (SI)  RndMeth=Simplest
  Data Type Conversion4 : DataTypeConversion  OutDataTypeStr=dataType  RndMeth=Simplest
  Data Type Conversion5 : DataTypeConversion  OutDataTypeStr=dataType  RndMeth=Simplest
  Data Type Conversion6 : DataTypeConversion  OutDataTypeStr=boolean
  Data_Conditioning : Subsystem
  Demux : Demux  Outputs=2
  Enable : Constant  OutDataTypeStr=single
  IqRef_current_to_PU : Gain  Gain=1/PU_System_motor2.I_base  RndMeth=Simplest  OutDataTypeStr=Inherit: Same as input
  Iq_Ref(A) : Step  Time=3  Before=1  After=0.8*pmsm_motor2.I_rated  OutDataTypeStr=single
  Mux : Mux  Inputs=2
  Speed_Ref_CW (rpm) : Step  Before=0.2*pmsm_motor1.N_base  After=0.5*pmsm_motor1.N_base  OutDataTypeStr=single
  rpm2PU : Gain  Gain=1/pmsm_motor1.N_base  RndMeth=Simplest  OutDataTypeStr=Inherit: Same as input
  Enable_PWM : Outport
  wires:
  Data Type Conversion3/1 -> Data_Conditioning/1(In1)
  rpm2PU/1 -> Data Type Conversion2/1
  Data Type Conversion1/1 -> Mux/2
  Data Type Conversion2/1 -> Mux/1
  Data Type Conversion/1 -> Data Type Conversion3/1
  Mux/1 -> Data Type Conversion/1
  Speed_Ref_CW (rpm)/1 -> rpm2PU/1
  IqRef_current_to_PU/1 -> Data Type Conversion1/1
  Iq_Ref(A)/1 -> IqRef_current_to_PU/1
  Data_Conditioning/1(Out1) -> Demux/1
  Demux/1 -> Data Type Conversion5/1
  Data Type Conversion4/1 -> Data Store Write2/1
  Demux/2 -> Data Type Conversion4/1
  Data Type Conversion5/1 -> Data Sore Write2/1
  Data Type Conversion6/1 -> Enable_PWM/1
  Enable/1 -> Data Type Conversion6/1

== system mcb_pmsm_foc_qep_dyno_f28069m_RAMP_ON_TARGET_R2021b/Simulation/Simulation1 ==
  Trigger : TriggerPort  VariantControl=Variant  PortDimensions=1
  ADCINT1 : simulink/Ports & Subsystems/Function-Call Generator  sample_time=-1  numberOfIterations=1  DisallowWideOutput=off
  Interrupt : Outport
  wires:
  ADCINT1/1 -> Interrupt/1

== system mcb_pmsm_foc_qep_dyno_f28069m_RAMP_ON_TARGET_R2021b/Simulation/Simulation2 ==
  Trigger : TriggerPort  VariantControl=Variant  PortDimensions=1
  ADCINT1 : simulink/Ports & Subsystems/Function-Call Generator  sample_time=-1  numberOfIterations=1  DisallowWideOutput=off
  Interrupt : Outport
  wires:
  ADCINT1/1 -> Interrupt/1

== system mcb_pmsm_foc_qep_dyno_f28069m_RAMP_ON_TARGET_R2021b/Speed Control for motor1/PI_Controller_Speed ==
  N_ref : Inport
  N_fb : Inport  Port=2
  AND : Logic  IconShape=distinctive  AllPortsSameDT=off  OutDataTypeStr=boolean
  Data Store Read1 : DataStoreRead  DataStoreName=Enable  IndexOptions=Index vector (dialog)  Indices=1  OutputSizes=1
  Data Store Read2 : DataStoreRead  DataStoreName=EnClosedLoop  IndexOptions=Index vector (dialog)  Indices=1  OutputSizes=1
  Discrete PI Controller with anti-windup & reset : slpidlib/PID Controller  Controller=PI  Form=Parallel  TimeDomain=Discrete-time  UseExternalTs=off  SampleTime=-1  IntegratorMethod=Forward Euler  FilterMethod=Forward Euler  ControllerParametersSource=external  P=1  I=1  D=0  N=100  UseFilter=on  TunerSelectOption=Transfer Function Based (PID Tuner App)  InitialConditionSource=external  InitialConditionForIntegrator=0  InitialConditionForFilter=0  DifferentiatorICPrevScaledInput=0  ExternalReset=level  TrackingMode=off  Kt=1  LimitOutput=on  SatLimitsSource=internal  UpperSaturationLimit=1  LowerSaturationLimit=-1  LinearizeAsGain=on  AntiWindupMode=clamping  Kb=1  RndMeth=Simplest  POutMin=[]  POutMax=[]  IOutMin=[]  IOutMax=[]  DOutMin=[]  DOutMax=[]  NOutMin=[]  NOutMax=[]  SumOutMin=[]  SumOutMax=[]  SaturationOutDataTypeStr=Inherit: Inherit via back propagation  SaturationOutMin=[]  SaturationOutMax=[]  PParamMin=[]  PParamMax=[]  IParamMin=[]  IParamMax=[]  DParamMin=[]  DParamMax=[]  NParamMin=[]  NParamMax=[]  KbParamMin=[]  KbParamMax=[]  KtParamMin=[]  KtParamMax=[]  KbOutMin=[]  KbOutMax=[]  KtOutMin=[]  KtOutMax=[]  IntegratorOutMin=[]  IntegratorOutMax=[]  FilterOutMin=[]  FilterOutMax=[]  SumI1OutMin=[]  SumI1OutMax=[]  SumI2OutMin=[]  SumI2OutMax=[]  SumI3OutMin=[]  SumI3OutMax=[]  SumI4OutMin=[]  SumI4OutMax=[]  SumDOutMin=[]  SumDOutMax=[]  DifferentiatorOutMin=[]  DifferentiatorOutMax=[]  FilterDiffOutCoefMin=[]  FilterDiffOutCoefMax=[]  ReciprocalOutMin=[]  ReciprocalOutMax=[]  SumDenOutMin=[]  SumDenOutMax=[]  SumNumOutMin=[]  SumNumOutMax=[]  DivideOutMin=[]  DivideOutMax=[]  UdiffTsProdOutMin=[]  UdiffTsProdOutMax=[]  NTsProdOutMin=[]  NTsProdOutMax=[]  UintegralTsProdOutMin=[]  UintegralTsProdOutMax=[]  UngainTsProdOutMin=[]  UngainTsProdOutMax=[]  IntegratorContinuousStateAttributes=''  IntegratorStateMustResolveToSignalObject=off  IntegratorRTWStateStorageClass=Auto  FilterContinuousStateAttributes=''  FilterStateMustResolveToSignalObject=off  FilterRTWStateStorageClass=Auto  ParallelPVariant=ExternalParameters  IdealPVariant=Disabled  IVariant=ExternalParameters  DVariant=Disabled  IntegratorVariant=Discrete  SatVariant=Enabled  AWVariant=DiscClampingParallel  PCopyVariant=Disabled  TRVariant=Disabled  FdbkBlocksVariant=Forward  IdealPFdbkVariant=Disabled  SatFdbkVariant=Disabled  DerivativeFilterVariant=Disabled  NVariant=Disabled  NCopyVariant=Disabled_SignalSpec  FilterICVariant=Disabled  IntegratorICVariant=ExternalICs  ExternalResetVariant=ExternalReset  TRSumVariant=Passthrough  SumFdbkVariant=Disabled  SumVariant=Sum_PI  TsampFilterVariant=InternalTs  TsampNgainVariant=Passthrough  TsampIntegralVariant=Disabled_SignalSpec  ExternalSaturationOutDataTypeStr=Inherit: Same as second input
  Ki1 : Constant  Value=PI_params_motor1.Ki_speed*Ts_speed  OutDataTypeStr=dataType  SampleTime=-1
  Ki2 : Constant  Value=0  OutDataTypeStr=dataType  SampleTime=-1
  Kp1 : Constant  Value=PI_params_motor1.Kp_speed  OutDataTypeStr=dataType  SampleTime=-1
  Logical Operator : Logic  Operator=NOT  IconShape=distinctive  AllPortsSameDT=off  OutDataTypeStr=boolean
  Sum : Sum  Inputs=|+-  OutDataTypeStr=Inherit: Same as first input
  Iq_ref : Outport  VectorParamsAs1DForOutWhenUnconnected=off
  wires:
  Discrete PI Controller with anti-windup & reset/1 -> Iq_ref/1
  Ki1/1 -> Discrete PI Controller with anti-windup & reset/3
  Kp1/1 -> Discrete PI Controller with anti-windup & reset/2
  N_fb/1 -> Sum/2
  N_ref/1 -> Sum/1
  Sum/1 -> Discrete PI Controller with anti-windup & reset/1
  Logical Operator/1 -> Discrete PI Controller with anti-windup & reset/4
  Ki2/1 -> Discrete PI Controller with anti-windup & reset/5
  AND/1 -> Logical Operator/1
  Data Store Read1/1 -> AND/1
  Data Store Read2/1 -> AND/2

== system mcb_pmsm_foc_qep_dyno_f28069m_RAMP_ON_TARGET_R2021b/Speed Control for motor1/Speed_Ref_Selector ==
  Speed_Ref_In : Inport
  Speed_Ref_Open : Inport  Port=2
  Data Store Read : DataStoreRead  DataStoreName=EnClosedLoop  IndexOptions=Index vector (dialog)  Indices=1  OutputSizes=1
  IIR Filter : mcbcontrolslib/IIR Filter  VariantControl=Low Pass Filter  VariantSelect=Low-pass  Filter_constant=0.01  advancedSettings=off  Ts=50e-6  cutOff_freq=32.1525
  Switch : Switch  Criteria=u2 > Threshold  Threshold=0.5
  Speed_Ref_PU : Outport
  wires:
  IIR Filter/1 -> Speed_Ref_PU/1
  Switch/1 -> IIR Filter/1
  Data Store Read/1 -> Switch/2
  Speed_Ref_Open/1 -> Switch/3
  Speed_Ref_In/1 -> Switch/1

== system mcb_pmsm_foc_qep_dyno_f28069m_RAMP_ON_TARGET_R2021b/FOC Algorithm Motor1/Control_System/Closed loop Control ==
  Iab_meas_PU : Inport
  Pos_PU : Inport  Port=2
  Idq_ref_PU : Inport  Port=3
  EnablePWM : Inport  Port=4
  Enable : EnablePort
  Current Control : Subsystem  ReferencedSubsystem=current_control  Kpd=PI_params_motor1.Kp_i  Kid=PI_params_motor1.Ki_i*Ts  Kpq=PI_params_motor1.Kp_i  Kiq=PI_params_motor1.Ki_i*Ts
  Terminator : Terminator
  Vabc in PU : Outport
  Idq_debug : Outport  Port=2
  wires:
  Current Control/1 -> Vabc in PU/1
  Idq_ref_PU/1 -> Current Control/3
  EnablePWM/1 -> Current Control/4
  Current Control/2 -> Idq_debug/1
  Pos_PU/1 -> Current Control/2
  Iab_meas_PU/1 -> Current Control/1
  Current Control/3 -> Terminator/1

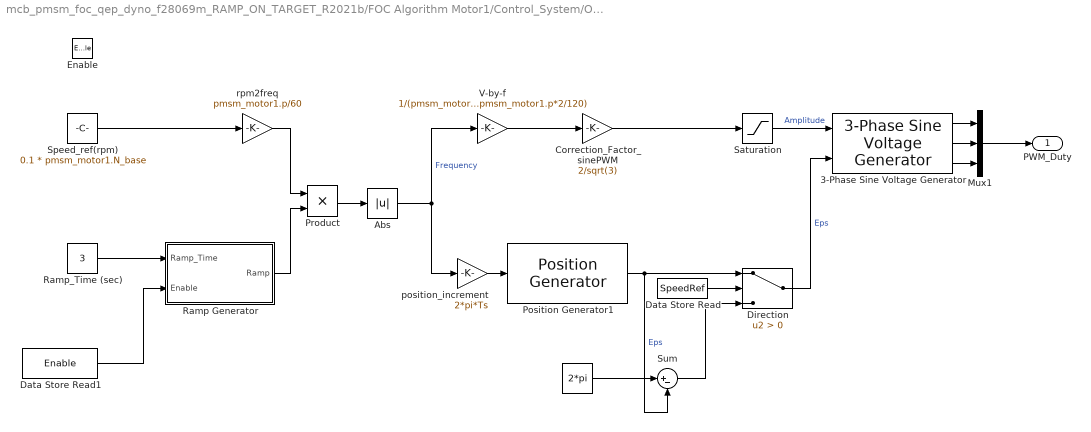
== system mcb_pmsm_foc_qep_dyno_f28069m_RAMP_ON_TARGET_R2021b/FOC Algorithm Motor1/Control_System/Open Loop Start-Up ==
  Enable : EnablePort
  " " : Constant  Value=2*pi  OutDataTypeStr=dataType  SampleTime=-1
  3-Phase Sine Voltage Generator : mcbcontrolslib/3-Phase Sine Voltage Generator  AngleInput=Radians  N_points=1024
  Abs : Abs
  Correction_Factor_sinePWM : Gain  Gain=2/sqrt(3)  RndMeth=Simplest  OutDataTypeStr=Inherit: Same as input
  Data Store Read : DataStoreRead  DataStoreName=SpeedRef  IndexOptions=Index vector (dialog)  Indices=1  OutputSizes=1
  Data Store Read1 : DataStoreRead  DataStoreName=Enable  IndexOptions=Index vector (dialog)  Indices=1  OutputSizes=1
  Direction : Switch  Criteria=u2 > Threshold  OutDataTypeStr=dataType  RndMeth=Simplest
  Mux1 : Mux  Inputs=3
  Position Generator1 : mcbcontrolslib/Position Generator  AngleOutput=Radians  ExternalReset=none  Offset=0
  Product : Product  RndMeth=Simplest  OutDataTypeStr=Inherit: Same as first input
  Ramp Generator : Subsystem
  Ramp_Time (sec) : Constant  Value=3  OutDataTypeStr=dataType  SampleTime=-1
  Saturation : Saturate  UpperLimit=0.95  LowerLimit=0.15  RndMeth=Simplest
  Speed_ref(rpm) : Constant  Value=0.1 * pmsm_motor1.N_base  OutDataTypeStr=dataType  SampleTime=-1
  Sum : Sum  Inputs=|+-  RndMeth=Simplest  OutDataTypeStr=Inherit: Same as first input
  V-by-f : Gain  Gain=1/(pmsm_motor1.N_base*pmsm_motor1.p*2/120)  RndMeth=Simplest  OutDataTypeStr=Inherit: Same as input
  position_increment : Gain  Gain=2*pi*Ts  RndMeth=Simplest  OutDataTypeStr=Inherit: Same as input
  rpm2freq : Gain  Gain=pmsm_motor1.p/60  RndMeth=Simplest  OutDataTypeStr=Inherit: Same as input
  PWM_Duty : Outport  VectorParamsAs1DForOutWhenUnconnected=off
  wires:
  3-Phase Sine Voltage Generator/1 -> Mux1/1
  3-Phase Sine Voltage Generator/3 -> Mux1/3
  Direction/1 -> 3-Phase Sine Voltage Generator/2  "Eps"
  Speed_ref(rpm)/1 -> rpm2freq/1
  Saturation/1 -> 3-Phase Sine Voltage Generator/1  "Amplitude"
  Mux1/1 -> PWM_Duty/1
  Ramp Generator/1(Ramp) -> Product/2
  Ramp_Time (sec)/1 -> Ramp Generator/1(Ramp_Time)
  Position Generator1/1 -> Sum/2, Direction/1  "Eps"
  " "/1 -> Sum/1
  Sum/1 -> Direction/3
  Abs/1 -> position_increment/1, V-by-f/1  "Frequency"
  position_increment/1 -> Position Generator1/1
  V-by-f/1 -> Correction_Factor_sinePWM/1
  Product/1 -> Abs/1
  rpm2freq/1 -> Product/1
  Correction_Factor_sinePWM/1 -> Saturation/1
  3-Phase Sine Voltage Generator/2 -> Mux1/2
  Data Store Read1/1 -> Ramp Generator/2(Enable)
  Data Store Read/1 -> Direction/2

== system mcb_pmsm_foc_qep_dyno_f28069m_RAMP_ON_TARGET_R2021b/FOC Algorithm Motor1/HW_Inputs/Sensor Driver Blocks (codegen) ==
  Sim : Inport
  IA/IB Measurement : c2802xlib/ADC  blkParamProc=C2000  ADCModule=1  samplingMode=Simultaneous sample mode  ADCResolution=12-bit (Single-ended input)  useSOC1=SOC0  useSOC2=SOC0_SOC1  SOCAcquisitionWindow=7  SOCTriggerSource=ePWM1_ADCSOCA  SOCInterruptTrigger=No ADCINT  Ts=-1  dType=uint16  postInterrupt=on  interruptSel=ADCINT1  ADCINTContinuous=on  endma=off  chdma=1  conv1=ADCINB1  conv2=ADCINA0 and ADCINB0  conv1_Type4=ADCIN0  conv2_Type4=ADCIN0 and ADCIN1
  Mux : Mux  Inputs=3
  Terminator : Terminator
  eQEP : c280xlib/eQEP  useModule=eQEP1  pcInputmode=Quadrature-count  externalClockrate=2x resolution: Count the rising/falling edge  swapPolarityselection=Clockwise  qdfOutputport=off  qapPolarityselection=on  qbpPolarityselection=on  qipPolarityselection=on  qspPolarityselection=off  igatePolarityselection=off  sampleTime=-1  pcOutputport=on  pcMaximumvalue=2^16-1  indexInitializationcheck=off  indexInitializationevent=Falling edge  strobeInitializationcheck=off  strobeInitializationevent=Rising edge  softwareInitializationcheck=off  softwareInitializationsource=Set to init value at start up  softwareInitializationmode=on  pcInitialvalue=0  pcResetmode=Reset on the first index event  ieloutputport=on  indexEventlatch=Falling edge  seloutputport=off  strobeEventlatch=Rising edge  pcefOutputport=off  enableEqepcapture=off  qctmrOutputport=off  qcprdOutputport=off  captureTimerprescaler=128  upEventprescaler=128  overflowErrorflag=off  directionErrorflag=off  captureTimerposition=On position counter read  unitTimerperiod=100000000  captureTimerlatch=off  capturePeriodlatch=off  positionCounterlatch=off  soenPolarityselection=off  spselPolarityselection=Index pin is used for sync output  compareValuesource=Specify via dialog  shadowMode=Load on QPOSCNT=0  compareValue=4294967295  syncOutputwidth=1  polaritySyncoutput=Active high  watchdogEnable=off  watchdogTimer=65535  outport1Datatype=auto  outport2Datatype=auto  outport3Datatype=auto  outport4Datatype=auto  outport5Datatype=auto  outport6Datatype=auto  outport7Datatype=auto  outport8Datatype=auto  outport9Datatype=auto  outport10Datatype=auto  outport11Datatype=auto  outport12Datatype=auto  eqepinterrupt_pce=off  eqepinterrupt_qpe=off  eqepinterrupt_qdc=off  eqepinterrupt_wto=off  eqepinterrupt_pcu=off  eqepinterrupt_pco=off  eqepinterrupt_pcr=off  eqepinterrupt_pcm=off  eqepinterrupt_sel=off  eqepinterrupt_iel=off  eqepinterrupt_uto=off  pheOutputport=off  watchdogOutputport=off  outport13Datatype=auto  outport14Datatype=auto
  out : Outport
  wires:
  Sim/1 -> Terminator/1
  Mux/1 -> out/1
  IA/IB Measurement/1 -> Mux/1
  eQEP/1 -> Mux/2
  eQEP/2 -> Mux/3

== system mcb_pmsm_foc_qep_dyno_f28069m_RAMP_ON_TARGET_R2021b/FOC Algorithm Motor1/HW_Inputs/Sensor Driver Blocks (sim) ==
  Sim : Inport
  out : Outport
  wires:
  Sim/1 -> out/1
